simulink model "LQR_FULL"  (R2013b)
settings: Solver=ode45  StartTime=0.0  StopTime=10.0  RelTol=1e-3
values from neighbouring files (symbols this model uses):
  b = 0.1    [QRLrunfile.m]    (also in hat.m = vec(2))
  ctauf = 8.004e-3    (= 0.008004)    [QRLrunfile.m]
  d = 0.1    [QRLrunfile.m]
  dq0 = [0;0;0]    [QRLrunfile.m]
  dxL0 = 0    [QRLrunfile.m]
  dyL0 = 0    [QRLrunfile.m]
  dzL0 = 0    [QRLrunfile.m]
  e3 = [0;0;1]    [QRLrunfile.m]
  fsat = inf*[1 -1]    [QRLrunfile.m]
  g = 9.81    [LQRrunfile.m]    (also in QRLrunfile.m)
  I = diag([Ixx Iyy Izz])    [QRLrunfile.m]
  Ir = 0.5    [QRLrunfile.m]
  Ixx = 0.0820    (= 0.082)    [LQRrunfile.m]    (also in QRLrunfile.m)
  Iyy = 0.0845    [LQRrunfile.m]    (also in QRLrunfile.m)
  Izz = 0.1377    [LQRrunfile.m]    (also in QRLrunfile.m)
  K = lqr(LQRA,LQRB,LQRQ,LQRR)    [LQRrunfile.m]
  l = 0.315    [QRLrunfile.m]
  lL = 0.7    [LQRrunfile.m]    (also in QRLrunfile.m)
  mL = 0.1    [LQRrunfile.m]    (also in QRLrunfile.m)
  mQ = 4.34    [LQRrunfile.m]    (also in QRLrunfile.m)
  Msat = inf*[1 -1]    [QRLrunfile.m]
  omega_n1_xL = 2*pi*.4    (= 2.51327412287)    [LQRrunfile.m]    (also in QRLrunfile.m)
  omega_n2_xL = 2*pi*.4    (= 2.51327412287)    [LQRrunfile.m]    (also in QRLrunfile.m = 3.45575191895)
  phiL0 = deg2rad(phiL0deg)    [QRLrunfile.m]
  pQ0 = 0    [QRLrunfile.m]
  psiL0 = 0    [QRLrunfile.m]
  q0 = [0 0 -1]    [QRLQRATT-18-Apr-2017.mat]    (also in QRLrunfile.m = Rzyx*e3*qmode; savename.mat)
  qQ0 = 0    [QRLrunfile.m]
  R0 = [1  0  0; 0  0.5  -0.866025403784; 0  0.866025403784  0.5]    [QRLQRATT-18-Apr-2017.mat]    (also in QRLrunfile.m = Rzyx; savename.mat)
  rQ0 = 0    [QRLrunfile.m]
  T0 = 3    [QRLrunfile.m]
  thetaL0 = deg2rad(thetaL0deg)    [QRLrunfile.m]
  xL0 = 0    [QRLrunfile.m]
  yL0 = 0    [QRLrunfile.m]
  zL0 = 0    [QRLrunfile.m]
undefined symbols (not defined in the file or in its folder): J, L, sigbuilder_block
libraries: simulink_extras x6, CF3 x5, simulink x5, vrlib x4, aerolibtransform2 x1
settings Model: Creator=Nam  LastModifiedBy=Nam

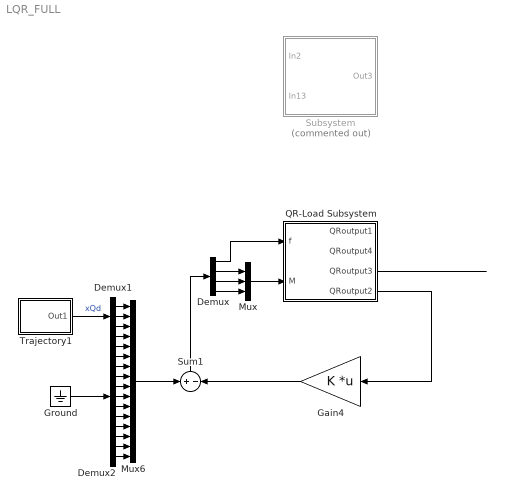
== system LQR_FULL ==
  Demux : Demux
  Demux1 : Demux  Outputs=3
  Demux2 : Demux  Outputs=13
  Gain4 : Gain  Gain=K  Multiplication=Matrix(K*u)
  Ground : Ground
  Mux : Mux  Inputs=3
  Mux6 : Mux  Inputs=16
  QR-Load Subsystem : Subsystem
  Subsystem : Subsystem  Commented=on
  Sum1 : Sum  Inputs=+|-
  Trajectory1 : Subsystem
  wires:
  QR-Load Subsystem/4(QRoutput2) -> Gain4/1
  Trajectory1/1(Out1) -> Demux1/1  "xQd"
  Demux1/1 -> Mux6/1
  Demux1/2 -> Mux6/2
  Demux1/3 -> Mux6/3
  Demux2/6 -> Mux6/9
  Demux2/11 -> Mux6/14
  Demux2/7 -> Mux6/10
  Demux2/10 -> Mux6/13
  Demux2/8 -> Mux6/11
  Demux2/12 -> Mux6/15
  Demux2/13 -> Mux6/16
  Demux2/5 -> Mux6/8
  Demux2/9 -> Mux6/12
  Demux2/4 -> Mux6/7
  Demux2/1 -> Mux6/4
  Demux2/2 -> Mux6/5
  Demux2/3 -> Mux6/6
  Ground/1 -> Demux2/1
  Mux6/1 -> Sum1/1
  Demux/1 -> QR-Load Subsystem/1(f)
  Mux/1 -> QR-Load Subsystem/2(M)
  Demux/2 -> Mux/1
  Demux/3 -> Mux/2
  Demux/4 -> Mux/3
  Sum1/1 -> Demux/1
  Gain4/1 -> Sum1/2
  QR-Load Subsystem/3(QRoutput3) -> ?

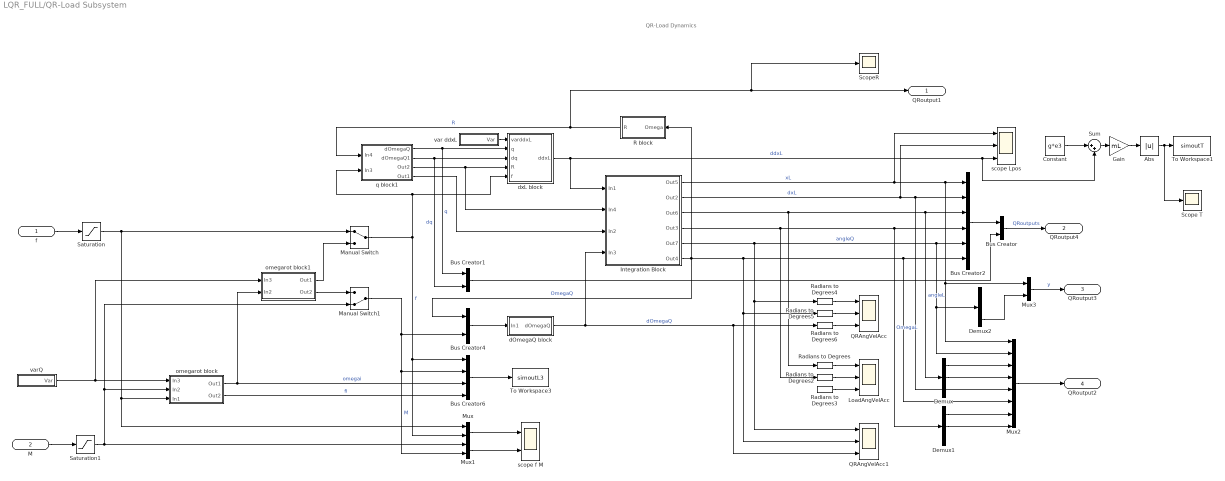
== system LQR_FULL/QR-Load Subsystem ==
  note: QR-Load Dynamics
  f : Inport
  M : Inport  Port=2  PortDimensions=3
  Abs : Abs
  Bus Creator : BusCreator  Inputs=2
  Bus Creator1 : BusCreator  Inputs=2
  Bus Creator2 : BusCreator  Inputs=6
  Bus Creator4 : BusCreator  Inputs=2
  Bus Creator6 : BusCreator
  Constant : Constant  Value=g*e3
  Demux : Demux  Outputs=3
  Demux1 : Demux  Outputs=3
  Demux2 : Demux  Outputs=3
  Gain : Gain  Gain=mL
  Integration Block : Subsystem
  LoadAngVelAcc : Scope  NumInputPorts=3
      settings: ShowLegends=on  YMin=-5~-5~-5  YMax=5~5~5  SaveName=ScopeData4
  Manual Switch : ManualSwitch
  Manual Switch1 : ManualSwitch  CurrentSetting=0
  Mux : Mux  Inputs=2
  Mux1 : Mux  Inputs=2
  Mux2 : Mux  Inputs=8
  Mux3 : Mux  Inputs=2
  QRAngVelAcc : Scope  NumInputPorts=3
      settings: ShowLegends=on  YMin=-40~-30~-600  YMax=20~30~600  SaveName=ScopeData3
  QRAngVelAcc1 : Scope  NumInputPorts=3
      settings: ShowLegends=on  YMin=-1~-20~-4000  YMax=5~45~4000  SaveName=ScopeData15
  R block : Subsystem
  Radians to Degrees{,2..6} (6 alike) : simulink_extras/Transformations/Radians to Degrees
  Saturation : Saturate  UpperLimit=fsat(1)  LowerLimit=fsat(2)
  Saturation1 : Saturate  UpperLimit=Msat(1)  LowerLimit=Msat(2)
  Scope T : Scope
      settings: YMin=0  YMax=15  SaveName=ScopeData43
  ScopeR : Scope
      settings: SaveName=ScopeData37
  Sum : Sum  Inputs=|++
  To Workspace1 : ToWorkspace  VariableName=simoutT  SampleTime=-1  SaveFormat=Structure With Time
  To Workspace3 : ToWorkspace  VariableName=simoutL3  SampleTime=-1  SaveFormat=Structure With Time
  dOmegaQ block : Subsystem
  dxL block : MATLAB Function  TreatAsAtomicUnit=on
  omegarot block : Subsystem
      mask Display: disp('(f,M) \rightarrow (\omega_i,f_i)','texmode','on')
  omegarot block1 : Subsystem
      mask Display: disp('sat(\omega_i) \rightarrow (f,M)','texmode','on')
  q block1 : Subsystem
  scope Lpos : Scope  NumInputPorts=3
      settings: ShowLegends=on  TimeRange=30  YMin=0~0~-100  YMax=7~6~250  SaveName=ScopeData12
  scope f M : Scope  NumInputPorts=2
      settings: ShowLegends=on  TimeRange=30  YMin=42~-4  YMax=54~5  SaveName=ScopeData42
  var ddxL : Subsystem
  varQ : Subsystem
  QRoutput1 : Outport
  QRoutput4 : Outport  Port=2
  QRoutput3 : Outport  Port=3
  QRoutput2 : Outport  Port=4
  wires:
  dxL block/1(ddxL) -> Sum/2, scope Lpos/3, Integration Block/1(In1)  "ddxL"
  dOmegaQ block/1(dOmegaQ) -> Integration Block/4(In3), Radians to Degrees6/1, QRAngVelAcc1/3  "dOmegaQ"
  Bus Creator4/1 -> dOmegaQ block/1(In1)
  M/1 -> Saturation1/1
  var ddxL/1(Var) -> dxL block/1(varddxL)
  q block1/2(dOmegaQ1) -> Bus Creator1/2, dxL block/3(dq)  "dq"
  q block1/3(Out2) -> Integration Block/2(In4), dxL block/4(R)
  q block1/1(dOmegaQ) -> Bus Creator1/1, dxL block/2(q)  "q"
  Integration Block/5(Out7) -> Demux2/1, Mux2/2, Bus Creator2/5, Radians to Degrees4/1, QRAngVelAcc1/1  "angleQ"
  Integration Block/2(Out2) -> Mux2/5, Bus Creator2/2, scope Lpos/2  "dxL"
  Integration Block/4(Out3) -> Demux1/1, Bus Creator2/4, Radians to Degrees2/1  "OmegaL"
  Integration Block/6(Out4) -> R block/1(Omega), Mux2/6, Bus Creator2/6, Radians to Degrees5/1, QRAngVelAcc1/2, Bus Creator4/1  "OmegaQ"
  Integration Block/1(Out5) -> Mux2/1, Mux3/1, Bus Creator2/1, scope Lpos/1  "xL"
  varQ/1(Var) -> omegarot block1/1(In3), omegarot block/1(In3)
  Integration Block/3(Out6) -> Bus Creator2/3, Demux/1, Radians to Degrees/1  "angleL"
  Bus Creator6/1 -> To Workspace3/1
  Radians to Degrees/1 -> LoadAngVelAcc/1
  Radians to Degrees2/1 -> LoadAngVelAcc/2
  Radians to Degrees3/1 -> LoadAngVelAcc/3
  Radians to Degrees5/1 -> QRAngVelAcc/2
  Radians to Degrees4/1 -> QRAngVelAcc/1
  Radians to Degrees6/1 -> QRAngVelAcc/3
  R block/1(R) -> q block1/1(In4), ScopeR/1, QRoutput1/1  "R"
  Bus Creator1/1 -> Bus Creator/2
  Bus Creator2/1 -> Bus Creator/1
  Bus Creator/1 -> QRoutput4/1  "QRoutputs"
  q block1/4(Out1) -> Integration Block/3(In2)
  f/1 -> Saturation/1
  Mux/1 -> scope f M/1
  Mux1/1 -> scope f M/2
  Constant/1 -> Sum/1
  Sum/1 -> Gain/1
  Gain/1 -> Abs/1
  Abs/1 -> Scope T/1, To Workspace1/1
  omegarot block/1(Out1) -> omegarot block1/2(In2), Bus Creator6/3  "omegai"
  Manual Switch/1 -> Bus Creator6/1, Mux/2, q block1/2(In3), dxL block/5(f)  "f"
  Manual Switch1/1 -> Bus Creator4/2, Bus Creator6/2, Mux1/2  "M"
  omegarot block1/1(Out1) -> Manual Switch/2
  Saturation/1 -> omegarot block/3(In1), Mux/1, Manual Switch/1
  Saturation1/1 -> Manual Switch1/2, omegarot block/2(In2), Mux1/1
  omegarot block/2(Out2) -> Bus Creator6/4  "fi"
  omegarot block1/2(Out2) -> Manual Switch1/1
  Mux2/1 -> QRoutput2/1
  Demux/1 -> Mux2/3
  Demux/2 -> Mux2/4
  Demux1/1 -> Mux2/7
  Demux1/2 -> Mux2/8
  Demux2/3 -> Mux3/2
  Mux3/1 -> QRoutput3/1  "y"

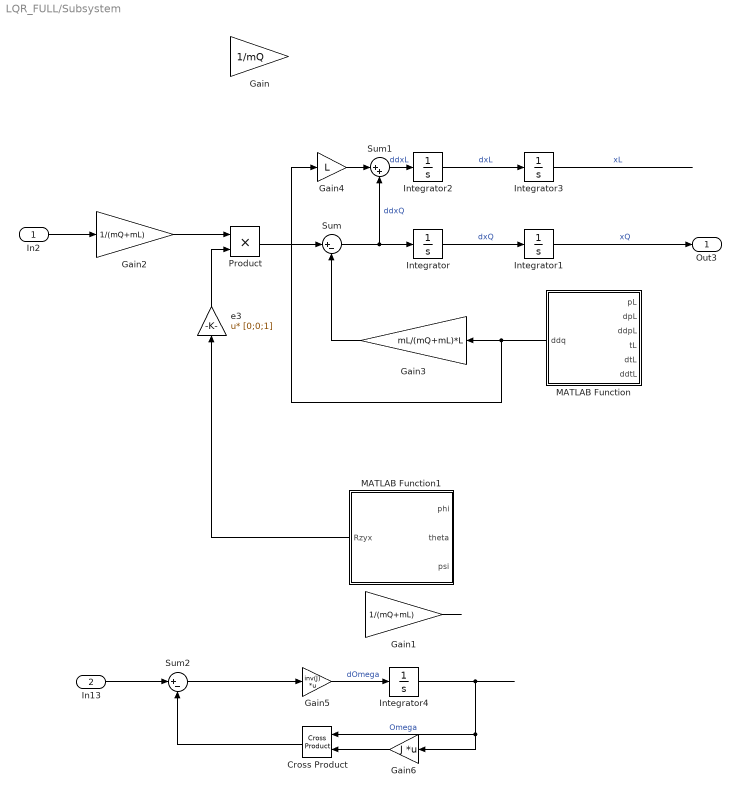
== system LQR_FULL/Subsystem ==
  In2 : Inport
  In13 : Inport  Port=2
  Cross Product : vrlib/Utilities/Cross Product
  Gain : Gain  Gain=1/mQ
  Gain1 : Gain  Gain=1/(mQ+mL)
  Gain2 : Gain  Gain=1/(mQ+mL)
  Gain3 : Gain  Gain=mL/(mQ+mL)*L
  Gain4 : Gain  Gain=L
  Gain5 : Gain  Gain=inv(J)  Multiplication=Matrix(K*u)
  Gain6 : Gain  Gain=J  Multiplication=Matrix(K*u)
  Integrator{,1..4} (5 alike) : Integrator
  MATLAB Function : MATLAB Function  TreatAsAtomicUnit=on
  MATLAB Function1 : MATLAB Function  TreatAsAtomicUnit=on
  Product : Product
  Sum : Sum  Inputs=|+-
  Sum1 : Sum  Inputs=|++
  Sum2 : Sum  Inputs=|+-
  e3 : Gain  Gain=[0;0;1]  Multiplication=Matrix(u*K)
  Out3 : Outport
  wires:
  e3/1 -> Product/2
  Integrator/1 -> Integrator1/1  "dxQ"
  Integrator1/1 -> Out3/1  "xQ"
  In13/1 -> Sum2/1
  Sum/1 -> Sum1/2, Integrator/1  "ddxQ"
  In2/1 -> Gain2/1
  ? -> MATLAB Function/6(ddtL)
  ? -> MATLAB Function/5(dtL)
  ? -> MATLAB Function/4(tL)
  ? -> MATLAB Function/3(ddpL)
  ? -> MATLAB Function/2(dpL)
  ? -> MATLAB Function/1(pL)
  ? -> MATLAB Function1/3(psi)
  ? -> MATLAB Function1/2(theta)
  ? -> MATLAB Function1/1(phi)
  Gain1/1 -> ?
  ? -> Gain1/1
  Gain3/1 -> Sum/2
  Gain2/1 -> Product/1
  Cross Product/1 -> Sum2/2
  Sum1/1 -> Integrator2/1  "ddxL"
  Sum2/1 -> Gain5/1
  Integrator2/1 -> Integrator3/1  "dxL"
  Gain6/1 -> Cross Product/2
  Gain5/1 -> Integrator4/1  "dOmega"
  Gain4/1 -> Sum1/1
  MATLAB Function/1(ddq) -> Gain4/1, Gain3/1
  Integrator4/1 -> Cross Product/1, Gain6/1  "Omega"
  Product/1 -> Sum/1
  Integrator3/1 -> ?  "xL"
  MATLAB Function1/1(Rzyx) -> e3/1

== system LQR_FULL/Trajectory1 ==
  Circle : Subsystem  Commented=on
  Manual Switch : ManualSwitch  CurrentSetting=0
  Manual Switch1 : ManualSwitch  CurrentSetting=0
  Path : Subsystem
  Step : Subsystem
  Out1 : Outport
  wires:
  Manual Switch1/1 -> Out1/1  "xLd"
  Manual Switch/1 -> Manual Switch1/2
  Circle/1(Out3) -> Manual Switch1/1
  Path/1(Out3) -> Manual Switch/1
  Step/1(Out2) -> Manual Switch/2

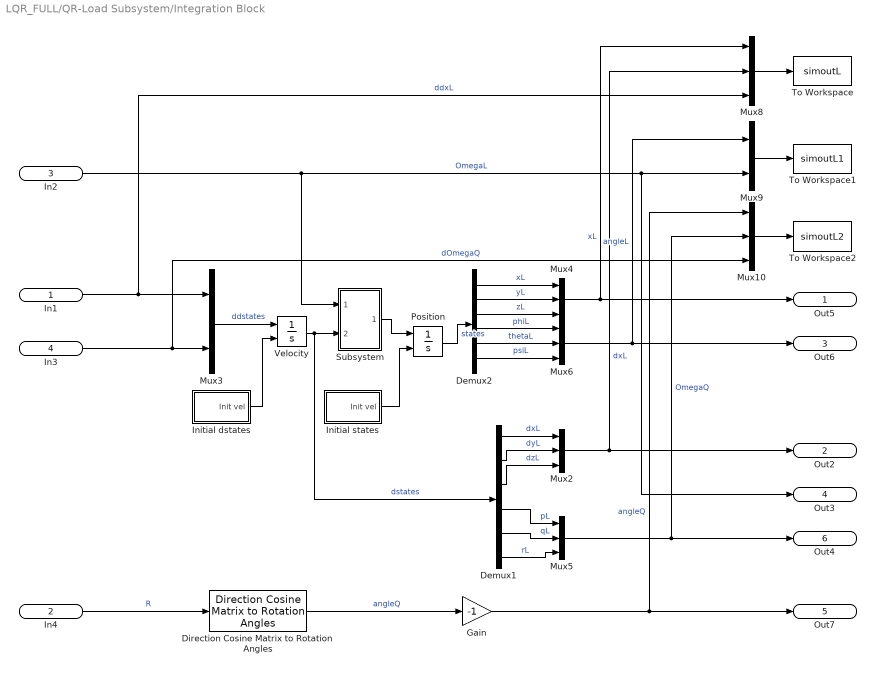
== system LQR_FULL/QR-Load Subsystem/Integration Block ==
  In1 : Inport
  In4 : Inport  Port=2
  In2 : Inport  Port=3
  In3 : Inport  Port=4
  Demux1 : Demux  Outputs=6
  Demux2 : Demux  Outputs=6
  Direction Cosine Matrix to Rotation Angles : aerolibtransform2/Direction Cosine Matrix to Rotation Angles  rotationOrder=XYZ  lim=Default
      settings: AttributesFormatString=Rotation Order: %<rotationOrder>
  Gain : Gain  Gain=-1
  Initial dstates : Subsystem
  Initial states : Subsystem
  Mux{2,4..6,8,10} (6 alike) : Mux  Inputs=3
  Mux3 : Mux  Inputs=2
  Mux9 : Mux  Inputs=2
  Position : Integrator  InitialConditionSource=external  ContinuousStateAttributes='position'
  Subsystem : Subsystem
  To Workspace : ToWorkspace  VariableName=simoutL  SampleTime=-1  SaveFormat=Structure With Time
  To Workspace1 : ToWorkspace  VariableName=simoutL1  SampleTime=-1  SaveFormat=Structure With Time
  To Workspace2 : ToWorkspace  VariableName=simoutL2  SampleTime=-1  SaveFormat=Structure With Time
  Velocity : Integrator  InitialConditionSource=external  ContinuousStateAttributes='velocity'
  Out5 : Outport
  Out2 : Outport  Port=2
  Out6 : Outport  Port=3
  Out3 : Outport  Port=4
  Out7 : Outport  Port=5
  Out4 : Outport  Port=6
  wires:
  In1/1 -> Mux8/3, Mux3/1  "ddxL"
  Demux1/2 -> Mux2/2  "dyL"
  Demux1/1 -> Mux2/1  "dxL"
  Demux1/3 -> Mux2/3  "dzL"
  Mux3/1 -> Velocity/1  "ddstates"
  Initial dstates/1(Init vel) -> Velocity/2
  Position/1 -> Demux2/1  "states"
  Demux2/2 -> Mux4/2  "yL"
  Demux2/1 -> Mux4/1  "xL"
  Demux2/3 -> Mux4/3  "zL"
  Initial states/1(Init vel) -> Position/2
  Demux2/4 -> Mux6/1  "phiL"
  Demux2/5 -> Mux6/2  "thetaL"
  Demux2/6 -> Mux6/3  "psiL"
  Velocity/1 -> Subsystem/2(In1), Demux1/1  "dstates"
  Mux2/1 -> Mux8/2, Out2/1  "dxL"
  Mux4/1 -> Mux8/1, Out5/1  "xL"
  In3/1 -> Mux3/2, Mux10/3  "dOmegaQ"
  Mux5/1 -> Mux10/2, Out4/1  "OmegaQ"
  Mux8/1 -> To Workspace/1
  Mux9/1 -> To Workspace1/1
  Mux10/1 -> To Workspace2/1
  Mux6/1 -> Out6/1, Mux9/1  "angleL"
  In2/1 -> Subsystem/1(In2), Mux9/2, Out3/1  "OmegaL"
  Subsystem/1(Out1) -> Position/1
  Demux1/5 -> Mux5/2  "qL"
  Demux1/6 -> Mux5/3  "rL"
  Demux1/4 -> Mux5/1  "pL"
  In4/1 -> Direction Cosine Matrix to Rotation Angles/1  "R"
  Direction Cosine Matrix to Rotation Angles/1 -> Gain/1  "angleQ"
  Gain/1 -> Mux10/1, Out7/1  "angleQ"

== system LQR_FULL/QR-Load Subsystem/R block ==
  note: R block
  Omega : Inport
  Integrator : Integrator  InitialCondition=R0  ContinuousStateAttributes='R'
  Saturation : Saturate  UpperLimit=1  LowerLimit=-1
  To Workspace4 : ToWorkspace  VariableName=simoutR  SampleTime=-1  SaveFormat=Structure With Time
  dR block : MATLAB Function  TreatAsAtomicUnit=on
  R : Outport
  wires:
  Integrator/1 -> Saturation/1  "R"
  dR block/1(dR) -> Integrator/1
  Omega/1 -> dR block/2(Omega)
  Saturation/1 -> dR block/1(R), To Workspace4/1, R/1  "R"

== system LQR_FULL/QR-Load Subsystem/dOmegaQ block ==
  In1 : Inport
  Add : Sum  Inputs=-+
  Bus Selector : BusSelector  OutputSignals=OmegaQ,M
  Gain2 : Gain  Gain=inv(I)  Multiplication=Matrix(K*u)
  Subsystem1 : Subsystem
      mask Display: disp('\Omega \times I\Omega','texmode','on')
  dOmegaQ : Outport
  wires:
  In1/1 -> Bus Selector/1  "varQ"
  Bus Selector/1 -> Subsystem1/1(Omega)  "<OmegaQ>"
  Subsystem1/1(Out1) -> Add/1
  Add/1 -> Gain2/1  "J*dOmega"
  Bus Selector/2 -> Add/2  "<M>"
  Gain2/1 -> dOmegaQ/1  "dOmegaQ"

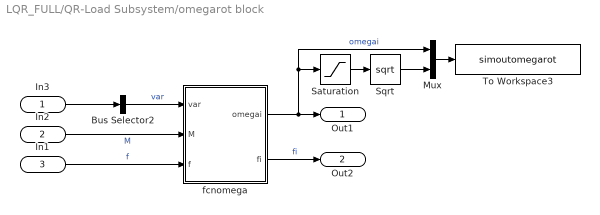
== system LQR_FULL/QR-Load Subsystem/omegarot block ==
  In3 : Inport
  In2 : Inport  Port=2
  In1 : Inport  Port=3
  Bus Selector2 : BusSelector  OutputSignals=sysvar.b,sysvar.d,sysvar.l  OutputAsBus=on
  Mux : Mux  Inputs=2
  Saturation : Saturate  UpperLimit=inf  LowerLimit=0  ZeroCross=off
  Sqrt : Sqrt  SaturateOnIntegerOverflow=on
  To Workspace3 : ToWorkspace  VariableName=simoutomegarot  SampleTime=-1  SaveFormat=Structure With Time
  fcnomega : MATLAB Function  TreatAsAtomicUnit=on
  Out1 : Outport
  Out2 : Outport  Port=2
  wires:
  In3/1 -> Bus Selector2/1
  In1/1 -> fcnomega/3(f)  "f"
  In2/1 -> fcnomega/2(M)  "M"
  Bus Selector2/1 -> fcnomega/1(var)  "var"
  Sqrt/1 -> Mux/2
  Saturation/1 -> Sqrt/1
  fcnomega/1(omegai) -> Mux/1, Saturation/1, Out1/1  "omegai"
  Mux/1 -> To Workspace3/1
  fcnomega/2(fi) -> Out2/1  "fi"

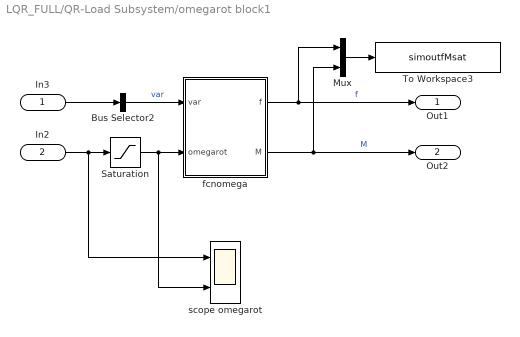
== system LQR_FULL/QR-Load Subsystem/omegarot block1 ==
  In3 : Inport
  In2 : Inport  Port=2
  Bus Selector2 : BusSelector  OutputSignals=sysvar.b,sysvar.d,sysvar.l  OutputAsBus=on
  Mux : Mux  Inputs=2
  Saturation : Saturate  UpperLimit=inf  LowerLimit=0  ZeroCross=off
  To Workspace3 : ToWorkspace  VariableName=simoutfMsat  SampleTime=-1  SaveFormat=Structure With Time
  fcnomega : MATLAB Function  TreatAsAtomicUnit=on
  scope omegarot : Scope  NumInputPorts=2
      settings: ShowLegends=on  TimeRange=2.154131847725163  YMin=-50~0  YMax=250~250  SaveName=ScopeData54
  Out1 : Outport
  Out2 : Outport  Port=2
  wires:
  In3/1 -> Bus Selector2/1
  In2/1 -> scope omegarot/1, Saturation/1
  Bus Selector2/1 -> fcnomega/1(var)  "var"
  fcnomega/1(f) -> Out1/1, Mux/1  "f"
  Mux/1 -> To Workspace3/1
  Saturation/1 -> scope omegarot/2, fcnomega/2(omegarot)
  fcnomega/2(M) -> Mux/2, Out2/1  "M"

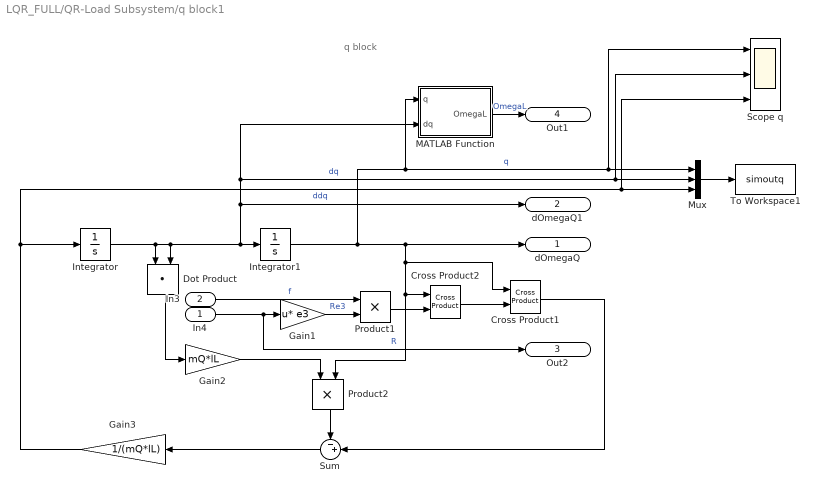
== system LQR_FULL/QR-Load Subsystem/q block1 ==
  note: q block
  In4 : Inport
  In3 : Inport  Port=2
  Cross Product1 : vrlib/Utilities/Cross Product
  Cross Product2 : vrlib/Utilities/Cross Product
  Dot Product : DotProduct  InputSameDT=on  OutDataTypeStr=Inherit: Inherit via internal rule
  Gain1 : Gain  Gain=e3  Multiplication=Matrix(u*K)
  Gain2 : Gain  Gain=mQ*lL
  Gain3 : Gain  Gain=1/(mQ*lL)
  Integrator : Integrator  InitialCondition=dq0  ContinuousStateAttributes='R'
  Integrator1 : Integrator  InitialCondition=q0  ContinuousStateAttributes='R'
  MATLAB Function : MATLAB Function  TreatAsAtomicUnit=on
  Mux : Mux  Inputs=3
  Product1 : Product
  Product2 : Product
  Scope q : Scope  NumInputPorts=3
      settings: ShowLegends=on  TimeRange=20  YMin=-1.2~-0.004~-0.006  YMax=0.2~0.002~0.006  SaveName=ScopeData39
  Sum : Sum  Inputs=-+|
  To Workspace1 : ToWorkspace  VariableName=simoutq  SampleTime=-1  SaveFormat=Structure With Time
  dOmegaQ : Outport
  dOmegaQ1 : Outport  Port=2
  Out2 : Outport  Port=3
  Out1 : Outport  Port=4
  wires:
  Dot Product/1 -> Gain2/1
  Gain3/1 -> Scope q/3, Mux/3, Integrator/1  "ddq"
  Integrator/1 -> Dot Product/1, Dot Product/2, Integrator1/1, dOmegaQ1/1, Scope q/2, Mux/2, MATLAB Function/2(dq)  "dq"
  In3/1 -> Product1/1  "f"
  Gain1/1 -> Product1/2  "Re3"
  Product1/1 -> Cross Product2/2
  Cross Product2/1 -> Cross Product1/2
  Cross Product1/1 -> Sum/2
  Sum/1 -> Gain3/1
  In4/1 -> Out2/1, Gain1/1  "R"
  Gain2/1 -> Product2/1
  Product2/1 -> Sum/1
  MATLAB Function/1(OmegaL) -> Out1/1  "OmegaL"
  Mux/1 -> To Workspace1/1
  Integrator1/1 -> dOmegaQ/1, Cross Product2/1, Product2/2, Cross Product1/1, Scope q/1, Mux/1, MATLAB Function/1(q)  "q"

== system LQR_FULL/QR-Load Subsystem/var ddxL ==
  Bus Creator1 : BusCreator
  Cable length : Constant  Value=lL
  Gravity Constant : Constant  Value=g
  Mass Load : Constant  Value=mL
  Mass QR : Constant  Value=mQ
  Var : Outport
  wires:
  Mass QR/1 -> Bus Creator1/1  "mQ"
  Cable length/1 -> Bus Creator1/4  "lL"
  Mass Load/1 -> Bus Creator1/3  "mL"
  Bus Creator1/1 -> Var/1  "varddxL"
  Gravity Constant/1 -> Bus Creator1/2  "g"

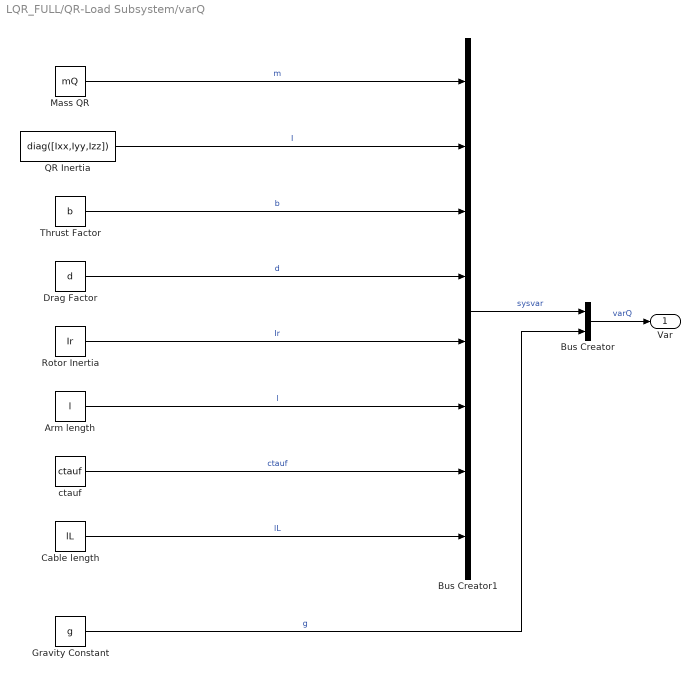
== system LQR_FULL/QR-Load Subsystem/varQ ==
  Arm length : Constant  Value=l
  Bus Creator : BusCreator  Inputs=2
  Bus Creator1 : BusCreator  Inputs=8
  Cable length : Constant  Value=lL
  Drag Factor : Constant  Value=d
  Gravity Constant : Constant  Value=g
  Mass QR : Constant  Value=mQ
  QR Inertia : Constant  Value=diag([Ixx,Iyy,Izz])
  Rotor Inertia : Constant  Value=Ir
  Thrust Factor : Constant  Value=b
  ctauf : Constant  Value=ctauf
      mask Display: disp('c_{\tau f}','texmode','on')
  Var : Outport
  wires:
  Gravity Constant/1 -> Bus Creator/2  "g"
  Bus Creator/1 -> Var/1  "varQ"
  Mass QR/1 -> Bus Creator1/1  "m"
  Arm length/1 -> Bus Creator1/6  "l"
  Rotor Inertia/1 -> Bus Creator1/5  "Ir"
  QR Inertia/1 -> Bus Creator1/2  "I"
  Bus Creator1/1 -> Bus Creator/1  "sysvar"
  Thrust Factor/1 -> Bus Creator1/3  "b"
  Drag Factor/1 -> Bus Creator1/4  "d"
  ctauf/1 -> Bus Creator1/7  "ctauf"
  Cable length/1 -> Bus Creator1/8  "lL"

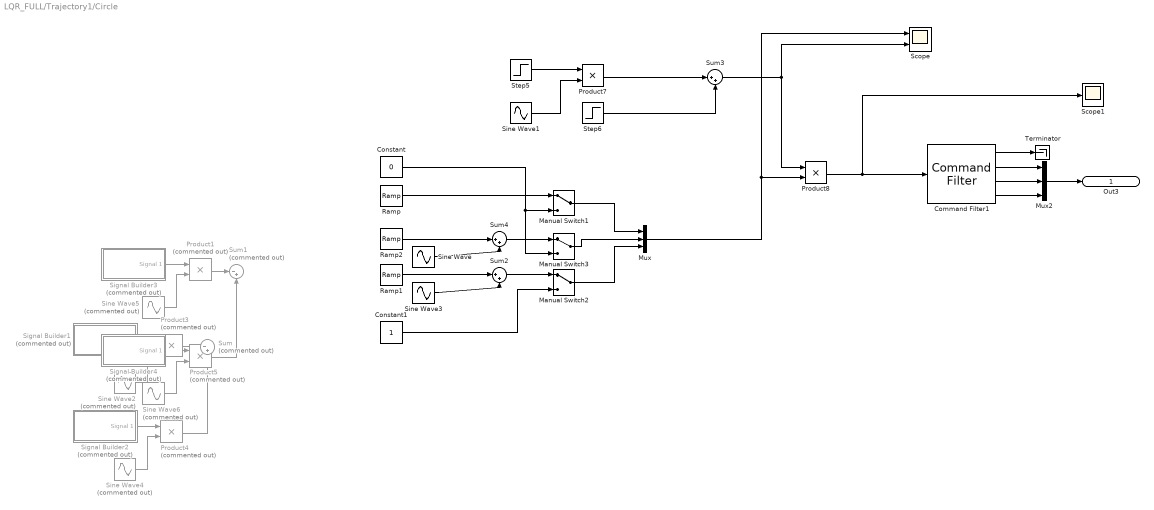
== system LQR_FULL/Trajectory1/Circle ==
  Command Filter1 : CF3/Command Filter  Integrator1_init=0  omega_n1=omega_n1_xL  omega_n2=omega_n2_xL  zeta=zeta_xL
  Constant : Constant  Value=0
  Constant1 : Constant
  Manual Switch1 : ManualSwitch
  Manual Switch2 : ManualSwitch
  Manual Switch3 : ManualSwitch
  Mux : Mux  Inputs=3
  Mux2 : Mux  Inputs=3
  Product{1,3..5} (4 alike) : Product  Commented=on
  Product7 : Product
  Product8 : Product
  Ramp : simulink/Sources/Ramp  slope=1/5  start=2  X0=0
  Ramp1 : simulink/Sources/Ramp  slope=0  start=0  X0=0
  Ramp2 : simulink/Sources/Ramp  slope=0  start=0  X0=0
  Scope : Scope  NumInputPorts=2
      settings: ShowLegends=on  YMin=-5~-5  YMax=5~5
  Scope1 : Scope
      settings: ShowLegends=on  YMin=-8  YMax=12  SaveName=ScopeData2
  Signal Builder1 : Subsystem  Tag=STV Subsys  Commented=on  LoadFcn=sigbuilder_block('load');  StartFcn=sigbuilder_block('start');  StopFcn=sigbuilder_block('stop');  ClipboardFcn=sigbuilder_block('clipboard');  mask(Sigbuilder block){}
      mask help: Simulink:masks:SigbuilderBlock_MD
      mask init:
      | if ~strcmp(get_param(bdroot(gcbh),'SimulationStatus'),'stopped') tuvar = sigbuilder_block('maskInit'); end
      settings: CopyFcn=sigbuilder_block('copy');  DeleteFcn=sigbuilder_block('delete');  ModelCloseFcn=sigbuilder_block('modelClose');  PreSaveFcn=sigbuilder_block('preSave');  PauseFcn=sigbuilder_block('pause');  ContinueFcn=sigbuilder_block('continue');  NameChangeFcn=sigbuilder_block('namechange');  OpenFcn=sigbuilder_block('open',[437.25 199.5 550.5 399.75 ]);  CloseFcn=sigbuilder_block('close');
      mask Display: plot(0, 0, 100, 100,[2, 2, 32, 32, 2], [68, 8, 8, 68, 68],[32, 2], [38, 38], [32, 19, 2],[53, 60, 44], [32, 17, 17, 2],[16, 16, 31, 31]);txt = getActiveGroup(gcbh);text(2, 100, txt,'verticalAlignment', 'top');
  Signal Builder2 : Subsystem  Tag=STV Subsys  Commented=on  LoadFcn=sigbuilder_block('load');  StartFcn=sigbuilder_block('start');  StopFcn=sigbuilder_block('stop');  ClipboardFcn=sigbuilder_block('clipboard');  mask(Sigbuilder block){}
      mask help: Simulink:masks:SigbuilderBlock_MD
      mask init:
      | if ~strcmp(get_param(bdroot(gcbh),'SimulationStatus'),'stopped') tuvar = sigbuilder_block('maskInit'); end
      settings: CopyFcn=sigbuilder_block('copy');  DeleteFcn=sigbuilder_block('delete');  ModelCloseFcn=sigbuilder_block('modelClose');  PreSaveFcn=sigbuilder_block('preSave');  PauseFcn=sigbuilder_block('pause');  ContinueFcn=sigbuilder_block('continue');  NameChangeFcn=sigbuilder_block('namechange');  OpenFcn=sigbuilder_block('open',[403.5 199.5 550.5 395.25 ]);  CloseFcn=sigbuilder_block('close');
      mask Display: plot(0, 0, 100, 100,[2, 2, 32, 32, 2], [68, 8, 8, 68, 68],[32, 2], [38, 38], [32, 19, 2],[53, 60, 44], [32, 17, 17, 2],[16, 16, 31, 31]);txt = getActiveGroup(gcbh);text(2, 100, txt,'verticalAlignment', 'top');
  Signal Builder3 : Subsystem  Tag=STV Subsys  Commented=on  LoadFcn=sigbuilder_block('load');  StartFcn=sigbuilder_block('start');  StopFcn=sigbuilder_block('stop');  ClipboardFcn=sigbuilder_block('clipboard');  mask(Sigbuilder block){}
      mask help: Simulink:masks:SigbuilderBlock_MD
      mask init:
      | if ~strcmp(get_param(bdroot(gcbh),'SimulationStatus'),'stopped') tuvar = sigbuilder_block('maskInit'); end
      settings: CopyFcn=sigbuilder_block('copy');  DeleteFcn=sigbuilder_block('delete');  ModelCloseFcn=sigbuilder_block('modelClose');  PreSaveFcn=sigbuilder_block('preSave');  PauseFcn=sigbuilder_block('pause');  ContinueFcn=sigbuilder_block('continue');  NameChangeFcn=sigbuilder_block('namechange');  OpenFcn=sigbuilder_block('open',[437.25 199.5 550.5 399.75 ]);  CloseFcn=sigbuilder_block('close');
      mask Display: plot(0, 0, 100, 100,[2, 2, 32, 32, 2], [68, 8, 8, 68, 68],[32, 2], [38, 38], [32, 19, 2],[53, 60, 44], [32, 17, 17, 2],[16, 16, 31, 31]);txt = getActiveGroup(gcbh);text(2, 100, txt,'verticalAlignment', 'top');
  Signal Builder4 : Subsystem  Tag=STV Subsys  Commented=on  LoadFcn=sigbuilder_block('load');  StartFcn=sigbuilder_block('start');  StopFcn=sigbuilder_block('stop');  ClipboardFcn=sigbuilder_block('clipboard');  mask(Sigbuilder block){}
      mask help: Simulink:masks:SigbuilderBlock_MD
      mask init:
      | if ~strcmp(get_param(bdroot(gcbh),'SimulationStatus'),'stopped') tuvar = sigbuilder_block('maskInit'); end
      settings: CopyFcn=sigbuilder_block('copy');  DeleteFcn=sigbuilder_block('delete');  ModelCloseFcn=sigbuilder_block('modelClose');  PreSaveFcn=sigbuilder_block('preSave');  PauseFcn=sigbuilder_block('pause');  ContinueFcn=sigbuilder_block('continue');  NameChangeFcn=sigbuilder_block('namechange');  OpenFcn=sigbuilder_block('open',[403.5 199.5 550.5 395.25 ]);  CloseFcn=sigbuilder_block('close');
      mask Display: plot(0, 0, 100, 100,[2, 2, 32, 32, 2], [68, 8, 8, 68, 68],[32, 2], [38, 38], [32, 19, 2],[53, 60, 44], [32, 17, 17, 2],[16, 16, 31, 31]);txt = getActiveGroup(gcbh);text(2, 100, txt,'verticalAlignment', 'top');
  Sine Wave : Sin  Amplitude=2.75  Frequency=2*pi/T0  Phase=-pi/2  SampleTime=0
  Sine Wave1 : Sin  Amplitude=0.5  Bias=0.5  Frequency=pi/(T0/2)  Phase=pi*1.5  SampleTime=0
  Sine Wave{2,4..6} (4 alike) : Sin  Commented=on  Amplitude=3  Frequency=2*pi/2.5  SampleTime=0
  Sine Wave3 : Sin  Frequency=2*pi/T0  SampleTime=0
  Step5 : Step  Time=(T0/2)  Before=1  After=0  SampleTime=0
  Step6 : Step  Time=(T0/2)  SampleTime=0
  Sum : Sum  Commented=on  Inputs=|-+
  Sum1 : Sum  Commented=on  Inputs=|-+
  Sum2 : Sum  Inputs=|++
  Sum3 : Sum  Inputs=|++
  Sum4 : Sum  Inputs=|++
  Terminator : Terminator
  Out3 : Outport
  wires:
  Constant/1 -> Manual Switch1/2, Manual Switch3/2
  Sine Wave3/1 -> Sum2/2
  Signal Builder1/1(Signal 1) -> Product3/1
  Sine Wave2/1 -> Product3/2
  Product3/1 -> Sum/1
  Signal Builder2/1(Signal 1) -> Product4/1
  Sine Wave4/1 -> Product4/2
  Product4/1 -> Sum/2
  Manual Switch3/1 -> Mux/2
  Manual Switch2/1 -> Mux/3
  Manual Switch1/1 -> Mux/1
  Mux/1 -> Product8/2, Scope/1
  Sine Wave1/1 -> Product7/2
  Step5/1 -> Product7/1
  Step6/1 -> Sum3/2
  Sum3/1 -> Product8/1, Scope/2
  Constant1/1 -> Manual Switch2/2
  Product7/1 -> Sum3/1
  Product8/1 -> Scope1/1, Command Filter1/1
  Signal Builder3/1(Signal 1) -> Product1/1
  Sine Wave5/1 -> Product1/2
  Product1/1 -> Sum1/1
  Signal Builder4/1(Signal 1) -> Product5/1
  Sine Wave6/1 -> Product5/2
  Product5/1 -> Sum1/2
  Ramp1/1 -> Sum2/1
  Ramp2/1 -> Sum4/1
  Sum4/1 -> Manual Switch3/1
  Sine Wave/1 -> Sum4/2
  Ramp/1 -> Manual Switch1/1
  Sum2/1 -> Manual Switch2/1
  Command Filter1/1 -> Terminator/1
  Command Filter1/3 -> Mux2/2
  Command Filter1/2 -> Mux2/1
  Command Filter1/4 -> Mux2/3
  Mux2/1 -> Out3/1

== system LQR_FULL/Trajectory1/Path ==
  CFP : CF3/Command Filter  Integrator1_init=0  omega_n1=omega_n1_xL*100  omega_n2=omega_n2_xL*50  zeta=zeta_xL
  Manual Switch : ManualSwitch
  Mux2 : Mux  Inputs=3
  Scope1 : Scope  NumInputPorts=3
      settings: TimeRange=25  YMin=-0.5~-0.8~-1.5  YMax=3.5~0.8~1.5  SaveName=ScopeData6
  Sine up down : Subsystem
  Square : Subsystem
  Terminator : Terminator
  Out3 : Outport
  wires:
  CFP/4 -> Scope1/3, Mux2/3
  CFP/3 -> Scope1/2, Mux2/2
  Manual Switch/1 -> CFP/1
  Square/1(Out1) -> Manual Switch/2
  Sine up down/1(Out2) -> Manual Switch/1
  CFP/1 -> Scope1/1, Out3/1, Mux2/1
  CFP/2 -> Terminator/1

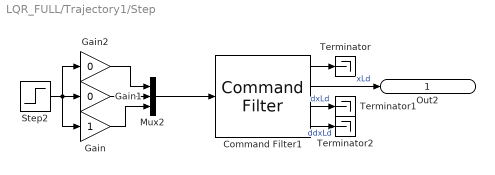
== system LQR_FULL/Trajectory1/Step ==
  Command Filter1 : CF3/Command Filter  Integrator1_init=0  omega_n1=2*pi*.75  omega_n2=2*pi*.75  zeta=.975
  Gain : Gain
  Gain1 : Gain  Gain=0
  Gain2 : Gain  Gain=0
  Mux2 : Mux  Inputs=3
  Step2 : Step  SampleTime=0
  Terminator : Terminator
  Terminator1 : Terminator
  Terminator2 : Terminator
  Out2 : Outport
  wires:
  Step2/1 -> Gain2/1, Gain/1, Gain1/1
  Mux2/1 -> Command Filter1/1
  Gain/1 -> Mux2/3
  Gain1/1 -> Mux2/2
  Gain2/1 -> Mux2/1
  Command Filter1/1 -> Terminator/1
  Command Filter1/2 -> Out2/1  "xLd"
  Command Filter1/3 -> Terminator1/1  "dxLd"
  Command Filter1/4 -> Terminator2/1  "ddxLd"

== system LQR_FULL/QR-Load Subsystem/Integration Block/Initial dstates ==
  Bus Creator1 : BusCreator  Inputs=2
  OmegaQ0 : Constant  Value=[pQ0; qQ0; rQ0]
  dxL0 : Constant  Value=[dxL0;dyL0;dzL0]
  Init vel : Outport
  wires:
  dxL0/1 -> Bus Creator1/1  "dxL0"
  Bus Creator1/1 -> Init vel/1  "Init dstates"
  OmegaQ0/1 -> Bus Creator1/2  "OmegaQ0"

== system LQR_FULL/QR-Load Subsystem/Integration Block/Initial states ==
  Bus Creator1 : BusCreator  Inputs=2
  angleL0 : Constant  Value=[phiL0; thetaL0; psiL0]
  xL0 : Constant  Value=[xL0;yL0;zL0]
  Init vel : Outport
  wires:
  xL0/1 -> Bus Creator1/1  "xL0"
  Bus Creator1/1 -> Init vel/1  "Init states"
  angleL0/1 -> Bus Creator1/2  "angleL0"

== system LQR_FULL/QR-Load Subsystem/Integration Block/Subsystem ==
  In2 : Inport
  In1 : Inport  Port=2
  Demux3 : Demux  Outputs=6
  Mux11 : Mux
  Out1 : Outport
  wires:
  Mux11/1 -> Out1/1
  In1/1 -> Demux3/1
  Demux3/2 -> Mux11/2
  Demux3/1 -> Mux11/1
  Demux3/3 -> Mux11/3
  In2/1 -> Mux11/4

== system LQR_FULL/QR-Load Subsystem/dOmegaQ block/Subsystem1 ==
  Omega : Inport
  Cross Product : vrlib/Utilities/Cross Product
  I : Gain  Gain=I  Multiplication=Matrix(K*u)
  Out1 : Outport
  wires:
  Omega/1 -> Cross Product/1, I/1
  I/1 -> Cross Product/2
  Cross Product/1 -> Out1/1

== system LQR_FULL/Trajectory1/Circle/Signal Builder1 ==
  Demux : Demux  Tag=STV Demux  Outputs=1
  FromWs : FromWorkspace  Tag=STV FromWs  VariableName=tuvar  SampleTime=0
      SigBuilderData=|
      | common.afterFinalStr = 'Extrapolate'
      | common.sampleTime = 0
      | dataSet.timeRange = [0 10]
      | dataSet.name = 'Group 1'
      | sbobj.Groups.Name = 'Group 1'
      | sbobj.Groups.Signals.Name = 'Signal 1'
      | sbobj.Groups.Signals.XData = [0 2.5 2.5 10]
      | sbobj.Groups.Signals.YData = [1 1 0 0]
  Signal 1 : Outport  Tag=STV Outport
  wires:
  Demux/1 -> Signal 1/1
  FromWs/1 -> Demux/1

== system LQR_FULL/Trajectory1/Circle/Signal Builder2 ==
  Demux : Demux  Tag=STV Demux  Outputs=1
  FromWs : FromWorkspace  Tag=STV FromWs  VariableName=tuvar  SampleTime=0
      SigBuilderData=|
      | common.afterFinalStr = 'Extrapolate'
      | common.sampleTime = 0
      | dataSet.timeRange = [0 10]
      | dataSet.name = 'Group 1'
      | sbobj.Groups.Name = 'Group 1'
      | sbobj.Groups.Signals.Name = 'Signal 1'
      | sbobj.Groups.Signals.XData = [0 2.5 2.5 5 5 10]
      | sbobj.Groups.Signals.YData = [0 0 1 1 0 0]
  Signal 1 : Outport  Tag=STV Outport
  wires:
  Demux/1 -> Signal 1/1
  FromWs/1 -> Demux/1

== system LQR_FULL/Trajectory1/Circle/Signal Builder3 ==
  Demux : Demux  Tag=STV Demux  Outputs=1
  FromWs : FromWorkspace  Tag=STV FromWs  VariableName=tuvar  SampleTime=0
      SigBuilderData=|
      | common.afterFinalStr = 'Extrapolate'
      | common.sampleTime = 0
      | dataSet.timeRange = [0 10]
      | dataSet.name = 'Group 1'
      | sbobj.Groups.Name = 'Group 1'
      | sbobj.Groups.Signals.Name = 'Signal 1'
      | sbobj.Groups.Signals.XData = [0 2.5 2.5 10]
      | sbobj.Groups.Signals.YData = [1 1 0 0]
  Signal 1 : Outport  Tag=STV Outport
  wires:
  FromWs/1 -> Demux/1
  Demux/1 -> Signal 1/1

== system LQR_FULL/Trajectory1/Circle/Signal Builder4 ==
  Demux : Demux  Tag=STV Demux  Outputs=1
  FromWs : FromWorkspace  Tag=STV FromWs  VariableName=tuvar  SampleTime=0
      SigBuilderData=|
      | common.afterFinalStr = 'Extrapolate'
      | common.sampleTime = 0
      | dataSet.timeRange = [0 10]
      | dataSet.name = 'Group 1'
      | sbobj.Groups.Name = 'Group 1'
      | sbobj.Groups.Signals.Name = 'Signal 1'
      | sbobj.Groups.Signals.XData = [0 2.5 2.5 5 5 10]
      | sbobj.Groups.Signals.YData = [0 0 1 1 0 0]
  Signal 1 : Outport  Tag=STV Outport
  wires:
  FromWs/1 -> Demux/1
  Demux/1 -> Signal 1/1

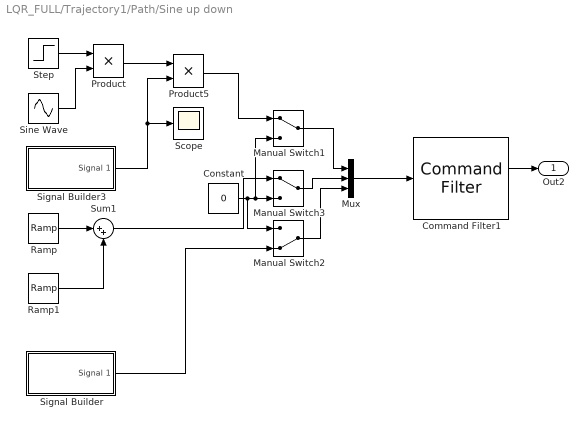
== system LQR_FULL/Trajectory1/Path/Sine up down ==
  Command Filter1 : CF3/Command Filter  Integrator1_init=0  omega_n1=omega_n1_xL  omega_n2=omega_n2_xL  zeta=zeta_xL
  Constant : Constant  Value=0
  Manual Switch1 : ManualSwitch
  Manual Switch2 : ManualSwitch  CurrentSetting=0
  Manual Switch3 : ManualSwitch
  Mux : Mux  Inputs=3
  Product : Product
  Product5 : Product
  Ramp : simulink/Sources/Ramp  slope=1/2  start=0  X0=0
  Ramp1 : simulink/Sources/Ramp  slope=-1/2  start=14  X0=0
  Scope : Scope
  Signal Builder : Subsystem  Tag=STV Subsys  LoadFcn=sigbuilder_block('load');  StartFcn=sigbuilder_block('start');  StopFcn=sigbuilder_block('stop');  ClipboardFcn=sigbuilder_block('clipboard');  mask(Sigbuilder block){}
      mask help: Simulink:masks:SigbuilderBlock_MD
      mask init:
      | if ~strcmp(get_param(bdroot(gcbh),'SimulationStatus'),'stopped') tuvar = sigbuilder_block('maskInit'); end
      settings: CopyFcn=sigbuilder_block('copy');  DeleteFcn=sigbuilder_block('delete');  ModelCloseFcn=sigbuilder_block('modelClose');  PreSaveFcn=sigbuilder_block('preSave');  PauseFcn=sigbuilder_block('pause');  ContinueFcn=sigbuilder_block('continue');  NameChangeFcn=sigbuilder_block('namechange');  OpenFcn=sigbuilder_block('open',[611.25 186.75 750 399.75 ]);  CloseFcn=sigbuilder_block('close');
      mask Display: plot(0, 0, 100, 100,[2, 2, 32, 32, 2], [68, 8, 8, 68, 68],[32, 2], [38, 38], [32, 19, 2],[53, 60, 44], [32, 17, 17, 2],[16, 16, 31, 31]);txt = getActiveGroup(gcbh);text(2, 100, txt,'verticalAlignment', 'top');
  Signal Builder3 : Subsystem  Tag=STV Subsys  LoadFcn=sigbuilder_block('load');  StartFcn=sigbuilder_block('start');  StopFcn=sigbuilder_block('stop');  ClipboardFcn=sigbuilder_block('clipboard');  mask(Sigbuilder block){}
      mask help: Simulink:masks:SigbuilderBlock_MD
      mask init:
      | if ~strcmp(get_param(bdroot(gcbh),'SimulationStatus'),'stopped') tuvar = sigbuilder_block('maskInit'); end
      settings: CopyFcn=sigbuilder_block('copy');  DeleteFcn=sigbuilder_block('delete');  ModelCloseFcn=sigbuilder_block('modelClose');  PreSaveFcn=sigbuilder_block('preSave');  PauseFcn=sigbuilder_block('pause');  ContinueFcn=sigbuilder_block('continue');  NameChangeFcn=sigbuilder_block('namechange');  OpenFcn=sigbuilder_block('open',[87.75 213.75 999 399.75 ]);  CloseFcn=sigbuilder_block('close');
      mask Display: plot(0, 0, 100, 100,[2, 2, 32, 32, 2], [68, 8, 8, 68, 68],[32, 2], [38, 38], [32, 19, 2],[53, 60, 44], [32, 17, 17, 2],[16, 16, 31, 31]);txt = getActiveGroup(gcbh);text(2, 100, txt,'verticalAlignment', 'top');
  Sine Wave : Sin  Amplitude=3  Frequency=2*pi/2.5  SampleTime=0
  Step : Step  Time=0  SampleTime=0
  Sum1 : Sum  Inputs=|++
  Out2 : Outport
  wires:
  Mux/1 -> Command Filter1/1
  Constant/1 -> Manual Switch3/2, Manual Switch1/2, Manual Switch2/1
  Manual Switch1/1 -> Mux/1
  Manual Switch2/1 -> Mux/3
  Ramp/1 -> Sum1/1
  Manual Switch3/1 -> Mux/2
  Step/1 -> Product/1
  Sine Wave/1 -> Product/2
  Product/1 -> Product5/1
  Product5/1 -> Manual Switch1/1
  Signal Builder3/1(Signal 1) -> Scope/1, Product5/2
  Ramp1/1 -> Sum1/2
  Sum1/1 -> Manual Switch3/1
  Signal Builder/1(Signal 1) -> Manual Switch2/2
  Command Filter1/2 -> Out2/1

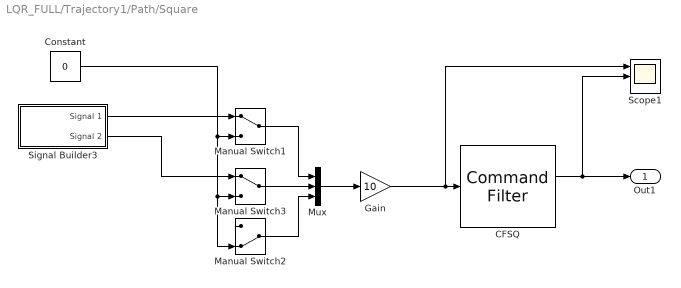
== system LQR_FULL/Trajectory1/Path/Square ==
  CFSQ : CF3/Command Filter  Integrator1_init=0  omega_n1=2*pi*1.2*0.5  omega_n2=2*pi*1*.5  zeta=zeta_xL
  Constant : Constant  Value=0
  Gain : Gain  Gain=10
  Manual Switch1 : ManualSwitch
  Manual Switch2 : ManualSwitch  CurrentSetting=0
  Manual Switch3 : ManualSwitch
  Mux : Mux  Inputs=3
  Scope1 : Scope  NumInputPorts=3
      settings: ShowLegends=on  TimeRange=15  YMin=0~0~-1  YMax=1~1~1  SaveName=ScopeData7
  Signal Builder3 : Subsystem  Tag=STV Subsys  LoadFcn=sigbuilder_block('load');  StartFcn=sigbuilder_block('start');  StopFcn=sigbuilder_block('stop');  ClipboardFcn=sigbuilder_block('clipboard');  mask(Sigbuilder block){}
      mask help: Simulink:masks:SigbuilderBlock_MD
      mask init:
      | if ~strcmp(get_param(bdroot(gcbh),'SimulationStatus'),'stopped') tuvar = sigbuilder_block('maskInit'); end
      settings: CopyFcn=sigbuilder_block('copy');  DeleteFcn=sigbuilder_block('delete');  ModelCloseFcn=sigbuilder_block('modelClose');  PreSaveFcn=sigbuilder_block('preSave');  PauseFcn=sigbuilder_block('pause');  ContinueFcn=sigbuilder_block('continue');  NameChangeFcn=sigbuilder_block('namechange');  OpenFcn=sigbuilder_block('open',[181.5 90.75 999 399.75 ]);  CloseFcn=sigbuilder_block('close');
      mask Display: plot(0, 0, 100, 100,[2, 2, 32, 32, 2], [68, 8, 8, 68, 68],[32, 2], [38, 38], [32, 19, 2],[53, 60, 44], [32, 17, 17, 2],[16, 16, 31, 31]);txt = getActiveGroup(gcbh);text(2, 100, txt,'verticalAlignment', 'top');
  Out1 : Outport
  wires:
  Constant/1 -> Manual Switch2/2, Manual Switch3/2, Manual Switch1/2
  Manual Switch1/1 -> Mux/1
  Manual Switch2/1 -> Mux/3
  Manual Switch3/1 -> Mux/2
  Mux/1 -> Gain/1
  CFSQ/2 -> Scope1/2, Out1/1
  Signal Builder3/1(Signal 1) -> Manual Switch1/1
  Signal Builder3/2(Signal 2) -> Manual Switch3/1
  Gain/1 -> Scope1/1, CFSQ/1

== system LQR_FULL/Trajectory1/Path/Sine up down/Signal Builder ==
  Demux : Demux  Tag=STV Demux  Outputs=1
  FromWs : FromWorkspace  Tag=STV FromWs  VariableName=tuvar  SampleTime=0
      SigBuilderData=|
      | common.afterFinalStr = 'Extrapolate'
      | common.sampleTime = 0
      | dataSet.timeRange = [0 15]
      | dataSet.name = 'Group 1'
      | sbobj.Groups.Name = 'Group 1'
      | sbobj.Groups.Signals.Name = 'Signal 1'
      | sbobj.Groups.Signals.XData = [0 2 7.5 12.5 15]
      | sbobj.Groups.Signals.YData = [0 0 1 0 0]
      | sbobj.Groups.TimeRange = [0 15]
  Signal 1 : Outport  Tag=STV Outport
  wires:
  Demux/1 -> Signal 1/1
  FromWs/1 -> Demux/1

== system LQR_FULL/Trajectory1/Path/Sine up down/Signal Builder3 ==
  Demux : Demux  Tag=STV Demux  Outputs=1
  FromWs : FromWorkspace  Tag=STV FromWs  VariableName=tuvar  SampleTime=0
      SigBuilderData=|
      | common.afterFinalStr = 'Extrapolate'
      | common.sampleTime = 0
      | dataSet.timeRange = [0 20]
      | dataSet.name = 'Group 1'
      | sbobj.Groups.Name = 'Group 1'
      | sbobj.Groups.Signals.Name = 'Signal 1'
      | sbobj.Groups.Signals.XData = [0 4 10 14 20]
      | sbobj.Groups.Signals.YData = [0 1 1 0 0]
      | sbobj.Groups.TimeRange = [0 20]
  Signal 1 : Outport  Tag=STV Outport
  wires:
  Demux/1 -> Signal 1/1
  FromWs/1 -> Demux/1

== system LQR_FULL/Trajectory1/Path/Square/Signal Builder3 ==
  Demux : Demux  Tag=STV Demux  Outputs=2
  FromWs : FromWorkspace  Tag=STV FromWs  VariableName=tuvar  SampleTime=0
      SigBuilderData=|
      | common.afterFinalStr = 'Extrapolate'
      | common.sampleTime = 0
      | dataSet.timeRange = [0 20]
      | dataSet.name = 'Group 1'
      | sbobj.Groups.Name = 'Group 1'
      | sbobj.Groups.Signals(1).Name = 'Signal 1'
      | sbobj.Groups.Signals(1).XData = [0 1 5 9 13 20]
      | sbobj.Groups.Signals(1).YData = [0 0 1 1 0 0]
      | sbobj.Groups.Signals(2).Name = 'Signal 2'
      | sbobj.Groups.Signals(2).XData = [0 5 9 13 17 20]
      | sbobj.Groups.Signals(2).YData = [0 0 1 1 0 0]
      | sbobj.Groups.TimeRange = [0 20]
  Signal 1 : Outport  Tag=STV Outport
  Signal 2 : Outport  Tag=STV Outport  Port=2
  wires:
  Demux/1 -> Signal 1/1
  FromWs/1 -> Demux/1
  Demux/2 -> Signal 2/1

== matlab function LQR_FULL/Subsystem/MATLAB Function1 ==
  data: phi input; theta input; psi input; Rzyx output
function Rzyx = fcn(phi,theta,psi)
%#codegen

Rz         = [cos(psi) -sin(psi) 0;
                sin(psi) cos(psi) 0;
                0 0 1];
Ry         = [cos(theta) 0 sin(theta);
                0 1 0;
                -sin(theta) 0 cos(theta)];
Rx         = [1 0 0;
                0 cos(phi) -sin(phi);
                0 sin(phi) cos(phi)];
Rzyx       = (Rx*Ry*Rz);

== matlab function LQR_FULL/Subsystem/MATLAB Function ==
  data: pL input; ddq output; dpL input; ddpL input; tL input; dtL input; ddtL input
function ddq = fcn(pL,dpL,ddpL,tL,dtL,ddtL)
%pL=pLhi, 
% tL=tLhetLa, 
% q=unitLvectLor qr-tLo-load

ddq = [ddtL*cos(tL)*cos(pL)-dtL^2*sin(tL)*cos(pL)-2*dtL*dpL*cos(tL)*sin(pL)-dpL^2*sin(tL)*cos(pL)-ddpL*sin(tL)*s(pL);
    ddtL*cos(tL)*sin(pL)-sin(tL)*sin(pL)*(dpL^2+dtL^2)+2*dpL*dtL*cos(tL)*c(pL)+ddpL*sin(tL)*cos(pL);
    -ddtL*sin(tL)-dtL^2*cos(tL)];

== matlab function LQR_FULL/QR-Load Subsystem/R block/dR block ==
  data: R input size=[3 3]; dR output size=[3 3]; Omega input size=3
function dR = fcn(R,Omega)
%#codegen
p = Omega(1);
q = Omega(2);
r = Omega(3);

Omegahat = [0 -r  q;
            r  0 -p;
           -q  p  0];

dR = R*Omegahat;
% R1 = R;

== matlab function LQR_FULL/QR-Load Subsystem/omegarot block1/fcnomega ==
  data: var input; f output size=1; M output size=3; omegarot input size=4
function [f,M] = fcn(var,omegarot)
%omega = [omega_1^2;omega_2^2;omega_3^2;omega_4^2]

b = var(1);
d = var(2);
l = var(3);

% %check if Gamma is invertible?
% Gamma = [b b b b;0 -l*b 0 l*b;l*b 0 -l*b 0;-d d -d d];
% 
% QRinput = [f;M];

f = [b b b b]*omegarot;
M = [0 -l*b 0 l*b;l*b 0 -l*b 0;-d d -d d]*omegarot;

== matlab function LQR_FULL/QR-Load Subsystem/omegarot block/fcnomega ==
  data: var input; M input size=3; f input; omegai output size=4; fi output
function [omegai,fi] = fcn(var,M,f)
%omega = [omega_1^2;omega_2^2;omega_3^2;omega_4^2]

b = var(1);
d = var(2);
l = var(3);

%check if Gamma is invertible?
Gamma = [b b b b;0 -l*b 0 l*b;l*b 0 -l*b 0;-d d -d d];

QRinput = [f;M];

omegai = Gamma\QRinput;
fi = b*omegai;

== matlab function LQR_FULL/QR-Load Subsystem/dxL block ==
  data: varddxL input; q input size=3; dq input; ddxL output size=3; R input size=[3 3]; f input size=1
function ddxL = fcn(varddxL,q,dq,R,f)

mQ = varddxL(1);
g  = varddxL(2);
mL = varddxL(3);
lL = varddxL(4);

e3 = [0;0;1];



ddxL = ( ( (dot(q,(f*R*e3)) - mQ*lL*dot(dq,dq)) * q ) / (mQ+mL) ) - g*e3;

== matlab function LQR_FULL/QR-Load Subsystem/q block1/MATLAB Function ==
  data: q input; OmegaL output; dq input
function OmegaL = fcn(q,dq)
%#codegen

qhat = [0 -q(3) q(2);
        q(3) 0 -q(1);
        -q(2) q(1) 0];


OmegaL = qhat*dq;
